simulink model "Grua_MC_R2_FFLimitado_06102026"  (R2025b)
settings: Solver=ode23t  StartTime=0.0  StopTime=628  MaxStep=T_s  RelTol=1e-4
InitFcn:
  | addpath(fileparts(get_param('Grua_MC_R2_FFLimitado_06102026','FileName')),'-begin');
  | run(fullfile(fileparts(get_param('Grua_MC_R2_FFLimitado_06102026','FileName')),'definir_buses_variadores.m'));
  | run(fullfile(fileparts(get_param('Grua_MC_R2_FFLimitado_06102026','FileName')),'parametros_ganancias_cascada_29072026.m'));
  | run(fullfile(fileparts(get_param('Grua_MC_R2_FFLimitado_06102026','FileName')),'configurar_modelo_final_hmi.m'));
  | run(fullfile(fileparts(get_param('Grua_MC_R2_FFLimitado_06102026','FileName')),'configurar_parametros_variadores.m'));
  | 
  | 
  | 
  | 
  | 
  | 
  | 
  | Pvis.Ts_viz=.04;Pvis.enable=true;Pvis.keepFigureOnTerminate=true;Pvis.hmi.captureFolder='D:\AyCD\Chat\Proyecto_grua\Prueba_Completa_MC_20261007\corrida_09';Pvis.hmi.fastDiagnostic=false;Pvis.hmi.testDriver=@operador_dos_traslados_v4;Pvis.hmi.renderPeriod=.20;
StopFcn:
  | guardar_prueba_completa;
undefined symbols (not defined in the file): b_cx, b_cy, b_hb, b_hEb, b_heq, b_t, b_tb, b_teq, b_tw, b_wu, g, H_c, HMI, i_h, i_t, J_heq, J_teq, K_cy, K_tw, k_wu, L_h0, l_hi, M_c_profile, M_s, M_t, MC_FF, nLevels0, omega_hmRATED, r_hd, r_td, slotBlock, T_hbMax, T_hEbMax, T_hmMax, T_s, T_s1, T_tbMax, T_tmMax, tau_hm, tau_tm, traj_duration, traj_x_start, traj_x_target, v_hmaxLoaded, v_hmaxUnloaded, x_tmax, x_tmin, Y_c0, Y_t0, Zbase
libraries: simulink x1, aerolibanimutils x1
(part 3 of 5)

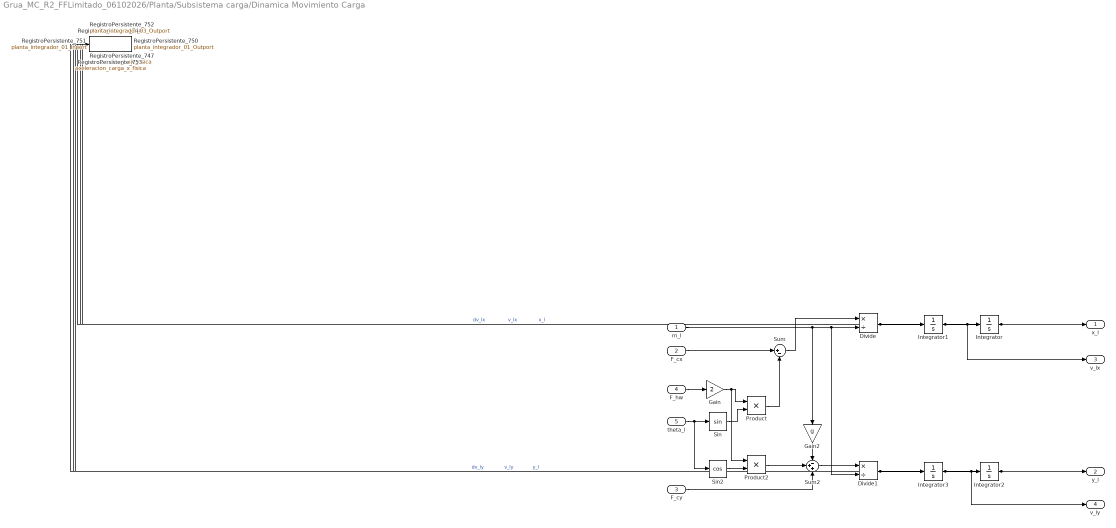
== system Grua_MC_R2_FFLimitado_06102026/Planta/Subsistema carga/Dinamica Movimiento Carga ==
  m_l : Inport
  F_cx : Inport  Port=2
  F_cy : Inport  Port=3
  F_hw : Inport  Port=4
  theta_l : Inport  Port=5
  Divide : Product  Inputs=*/
  Divide1 : Product  Inputs=*/
  Gain : Gain  Gain=2
  Gain2 : Gain  Gain=g
  Integrator : Integrator
  Integrator1 : Integrator
  Integrator2 : Integrator  InitialCondition=25
  Integrator3 : Integrator
  Product : Product
  Product2 : Product
  RegistroPersistente_746 : ToWorkspace  VariableName=diag_load_acc1  SaveFormat=Timeseries  SampleTime=-1
      settings: Decimation=10
  RegistroPersistente_747 : ToWorkspace  VariableName=aceleracion_izaje_fisica  SaveFormat=Timeseries  SampleTime=-1
      settings: Decimation=10
  RegistroPersistente_750 : ToWorkspace  VariableName=planta_integrador_01_Outport  SaveFormat=Timeseries  SampleTime=-1
      settings: Decimation=10
  RegistroPersistente_751 : ToWorkspace  VariableName=planta_integrador_01_Inport  SaveFormat=Timeseries  SampleTime=-1
      settings: Decimation=10
  RegistroPersistente_752 : ToWorkspace  VariableName=planta_integrador_03_Outport  SaveFormat=Timeseries  SampleTime=-1
      settings: Decimation=10
  RegistroPersistente_753 : ToWorkspace  VariableName=aceleracion_carga_x_fisica  SaveFormat=Timeseries  SampleTime=-1
      settings: Decimation=10
  Sin : Trigonometry
  Sin2 : Trigonometry  Operator=cos
  Sum : Sum  Inputs=|+-
  Sum2 : Sum  Inputs=-++
  x_l : Outport
  y_l : Outport  Port=2
  v_lx : Outport  Port=3
  v_ly : Outport  Port=4
  wires:
  Integrator/1 -> x_l/1, RegistroPersistente_750/1  "x_l"
  Integrator1/1 -> v_lx/1, Integrator/1, RegistroPersistente_751/1  "v_lx"
  Divide/1 -> Integrator1/1, RegistroPersistente_746/1  "dv_lx"
  Sum/1 -> Divide/1
  F_cx/1 -> Sum/1
  Gain/1 -> Product2/1, Product/1
  F_hw/1 -> Gain/1
  theta_l/1 -> Sin2/1, Sin/1
  Sin/1 -> Product/2
  Product/1 -> Sum/2
  Divide1/1 -> Integrator3/1, RegistroPersistente_747/1  "dv_ly"
  F_cy/1 -> Sum2/3
  m_l/1 -> Divide1/2, Divide/2, Gain2/1
  Integrator3/1 -> v_ly/1, Integrator2/1, RegistroPersistente_753/1  "v_ly"
  Integrator2/1 -> y_l/1, RegistroPersistente_752/1  "y_l"
  Sin2/1 -> Product2/2
  Product2/1 -> Sum2/2
  Gain2/1 -> Sum2/1
  Sum2/1 -> Divide1/1

== system Grua_MC_R2_FFLimitado_06102026/Planta/Subsistema carro/Dinamica Carro Traslacional ==
  F_tw : Inport
  F_hw : Inport  Port=2
  theta_l : Inport  Port=3
  Gain : Gain  Gain=1/M_t
  Gain1 : Gain  Gain=b_t
  Gain2 : Gain  Gain=2
  Integrator : Integrator
  Integrator1 : Integrator
  Product : Product
  RegistroPersistente_773 : ToWorkspace  VariableName=aceleracion_carro_fisica  SaveFormat=Timeseries  SampleTime=-1
      settings: Decimation=10
  RegistroPersistente_776 : ToWorkspace  VariableName=planta_integrador_05_Outport  SaveFormat=Timeseries  SampleTime=-1
      settings: Decimation=10
  RegistroPersistente_777 : ToWorkspace  VariableName=diag_xtrolley  SaveFormat=Timeseries  SampleTime=-1
      settings: Decimation=10
  Sin : Trigonometry
  Sum : Sum  Inputs=++-
  x_t : Outport
  v_t : Outport  Port=2
  wires:
  Sum/1 -> Gain/1
  Product/1 -> Gain2/1
  Gain/1 -> Integrator/1, RegistroPersistente_773/1  "ddx_t"
  Gain2/1 -> Sum/1  "ddx_t"
  Integrator1/1 -> x_t/1, RegistroPersistente_777/1  "x_t"
  F_tw/1 -> Sum/2
  Gain1/1 -> Sum/3
  Integrator/1 -> Gain1/1, v_t/1, Integrator1/1, RegistroPersistente_776/1  "v_t"
  Sin/1 -> Product/1
  F_hw/1 -> Product/2
  theta_l/1 -> Sin/1

== system Grua_MC_R2_FFLimitado_06102026/Planta/Subsistema carro/Dinamica Tambor Carro ==
  F_tw : Inport
  T_tm : Inport  Port=2
  T_tb : Inport  Port=3
  Gain3 : Gain  Gain=1/J_teq
  Gain4 : Gain  Gain=b_teq
  Gain5 : Gain  Gain=1/i_t
  Gain6 : Gain  Gain=r_td
  Gain7 : Gain  Gain=r_td
  Gain8 : Gain  Gain=r_td
  Integrator2 : Integrator
  Integrator3 : Integrator
  RegistroPersistente_788 : ToWorkspace  VariableName=planta_integrador_07_Inport  SaveFormat=Timeseries  SampleTime=-1
      settings: Decimation=10
  RegistroPersistente_792 : ToWorkspace  VariableName=diag_xdrum  SaveFormat=Timeseries  SampleTime=-1
      settings: Decimation=10
  RegistroPersistente_793 : ToWorkspace  VariableName=diag_vdrum  SaveFormat=Timeseries  SampleTime=-1
      settings: Decimation=10
  RegistroPersistente_794 : ToWorkspace  VariableName=planta_integrador_07_Outport  SaveFormat=Timeseries  SampleTime=-1
      settings: Decimation=10
  RegistroPersistente_795 : ToWorkspace  VariableName=planta_integrador_08_Outport  SaveFormat=Timeseries  SampleTime=-1
      settings: Decimation=10
  Sum1 : Sum  Inputs=++--
  x_td : Outport
  dx_td : Outport  Port=2
  theta_td : Outport  Port=3
  omega_td : Outport  Port=4
  wires:
  Gain3/1 -> Integrator2/1, RegistroPersistente_788/1  "ddtheta_td"
  Integrator2/1 -> omega_td/1, Gain4/1, Gain8/1, Integrator3/1, RegistroPersistente_794/1  "omega_td"
  Sum1/1 -> Gain3/1
  T_tb/1 -> Sum1/2
  Integrator3/1 -> Gain7/1, theta_td/1, RegistroPersistente_795/1  "theta_td"
  Gain6/1 -> Gain5/1  "T_tdl"
  Gain4/1 -> Sum1/4
  Gain5/1 -> Sum1/3  "ddtheta_td"
  T_tm/1 -> Sum1/1
  Gain7/1 -> x_td/1, RegistroPersistente_792/1  "x_td"
  Gain8/1 -> dx_td/1, RegistroPersistente_793/1  "dx_td"
  F_tw/1 -> Gain6/1

== system Grua_MC_R2_FFLimitado_06102026/Planta/Subsistema carro/Dinamica cable carro ==
  x_t : Inport
  dx_t : Inport  Port=2
  x_td : Inport  Port=3
  dx_td : Inport  Port=4
  Gain10 : Gain  Gain=b_tw
  Gain9 : Gain  Gain=K_tw
  Sum2 : Sum  Inputs=|+-
  Sum3 : Sum  Inputs=|+-
  Sum4 : Sum
  F_tw : Outport
  wires:
  x_t/1 -> Sum2/2
  Gain9/1 -> Sum4/1  "T_tdl"
  Sum4/1 -> F_tw/1  "F_tw"
  dx_t/1 -> Sum3/2
  dx_td/1 -> Sum3/1
  Sum2/1 -> Gain9/1
  Sum3/1 -> Gain10/1
  x_td/1 -> Sum2/1
  Gain10/1 -> Sum4/2  "T_tdl"

== system Grua_MC_R2_FFLimitado_06102026/Planta/Subsistema carro/Modelo Freno Operacion Carro ==
  BRK_t : Inport
  omega_tm : Inport  Port=2
  Constant : Constant  Value=0
  Gain : Gain  Gain=-b_tb
  RegistroPersistente_815 : ToWorkspace  VariableName=diag_brake_torque  SaveFormat=Timeseries  SampleTime=-1
      settings: Decimation=10
  Saturation : Saturate  UpperLimit=T_tbMax  LowerLimit=-T_tbMax
  Switch : Switch  Criteria=u2 > Threshold  SaturateOnIntegerOverflow=off  InputSameDT=off
  T_tb : Outport
  wires:
  Saturation/1 -> Switch/3
  omega_tm/1 -> Gain/1
  Switch/1 -> T_tb/1, RegistroPersistente_815/1
  Gain/1 -> Saturation/1
  Constant/1 -> Switch/1
  BRK_t/1 -> Switch/2

== system Grua_MC_R2_FFLimitado_06102026/Planta/Subsistema carro/Modulador de Torque Motor Drive Carro ==
  T_tm* : Inport
  Diferencia torque saturacion : Sum  Inputs=+-
  Gain : Gain  Gain=1/tau_tm
  Integrator : Integrator
  RegistroPersistente_819 : ToWorkspace  VariableName=aw_delta_torque_Nm  SaveFormat=Timeseries  SampleTime=-1
      settings: Decimation=10
  RegistroPersistente_820 : ToWorkspace  VariableName=planta_integrador_09_Inport  SaveFormat=Timeseries  SampleTime=-1
      settings: Decimation=10
  RegistroPersistente_821 : ToWorkspace  VariableName=planta_integrador_09_Outport  SaveFormat=Timeseries  SampleTime=-1
      settings: Decimation=10
  RegistroPersistente_822 : ToWorkspace  VariableName=torque_carro_limitado  SaveFormat=Timeseries  SampleTime=-1
      settings: Decimation=10
  Saturation : Saturate  UpperLimit=T_tmMax  LowerLimit=-T_tmMax
  Sum : Sum  Inputs=|+-
  T_tm : Outport
  Delta torque limite : Outport  Port=2
  wires:
  Integrator/1 -> Sum/2, T_tm/1, RegistroPersistente_821/1
  Gain/1 -> Integrator/1, RegistroPersistente_820/1
  Sum/1 -> Gain/1
  Saturation/1 -> Sum/1, Diferencia torque saturacion/1, RegistroPersistente_822/1  "T_tmlim*"
  T_tm*/1 -> Saturation/1, Diferencia torque saturacion/2
  Diferencia torque saturacion/1 -> Delta torque limite/1, RegistroPersistente_819/1

== system Grua_MC_R2_FFLimitado_06102026/Planta/Subsistema izaje/Calculo longitud l_h ==
  note: $\dot{l}_h(t)=-\frac{r_{hd}}{2}\omega_{hd}(t)$
  omega_hd : Inport
  Gain : Gain  Gain=-r_hd/2
  Integrator : Integrator  InitialCondition=l_hi
  RegistroPersistente_837 : ToWorkspace  VariableName=planta_integrador_10_Inport  SaveFormat=Timeseries  SampleTime=-1
      settings: Decimation=10
  RegistroPersistente_838 : ToWorkspace  VariableName=planta_integrador_10_Outport  SaveFormat=Timeseries  SampleTime=-1
      settings: Decimation=10
  l_h : Outport
  dl_h : Outport  Port=2
  wires:
  Integrator/1 -> l_h/1, RegistroPersistente_838/1  "l_h"
  omega_hd/1 -> Gain/1
  Gain/1 -> dl_h/1, Integrator/1, RegistroPersistente_837/1  "dl_h"

== system Grua_MC_R2_FFLimitado_06102026/Planta/Subsistema izaje/Dinamica Tambor Izaje ==
  T_hEb : Inport
  T_hm : Inport  Port=2
  F_hw : Inport  Port=3
  T_hb : Inport  Port=4
  Gain1 : Gain  Gain=r_hd
  Gain2 : Gain  Gain=1/i_h
  Gain3 : Gain  Gain=1/J_heq
  Gain4 : Gain  Gain=b_heq
  Gain5 : Gain  Gain=1/i_h
  Integrator2 : Integrator
  Integrator3 : Integrator
  RegistroPersistente_847 : ToWorkspace  VariableName=planta_integrador_11_Inport  SaveFormat=Timeseries  SampleTime=-1
      settings: Decimation=10
  RegistroPersistente_850 : ToWorkspace  VariableName=tambor_izaje_velocidad_angular  SaveFormat=Timeseries  SampleTime=-1
      settings: Decimation=10
  RegistroPersistente_851 : ToWorkspace  VariableName=planta_integrador_12_Outport  SaveFormat=Timeseries  SampleTime=-1
      settings: Decimation=10
  Sum1 : Sum  Inputs=+++--
  theta_hd : Outport
  omega_hd : Outport  Port=2
  wires:
  Gain3/1 -> Integrator2/1, RegistroPersistente_847/1  "ddtheta_hd"
  Integrator2/1 -> omega_hd/1, Gain4/1, Integrator3/1, RegistroPersistente_850/1  "omega_hd"
  Sum1/1 -> Gain3/1
  T_hb/1 -> Sum1/2
  T_hEb/1 -> Gain5/1  "T_hEb"
  Gain4/1 -> Sum1/5
  Gain5/1 -> Sum1/3
  T_hm/1 -> Sum1/1
  F_hw/1 -> Gain1/1
  Gain1/1 -> Gain2/1  "T_hdl"
  Gain2/1 -> Sum1/4
  Integrator3/1 -> theta_hd/1, RegistroPersistente_851/1  "theta_hd"

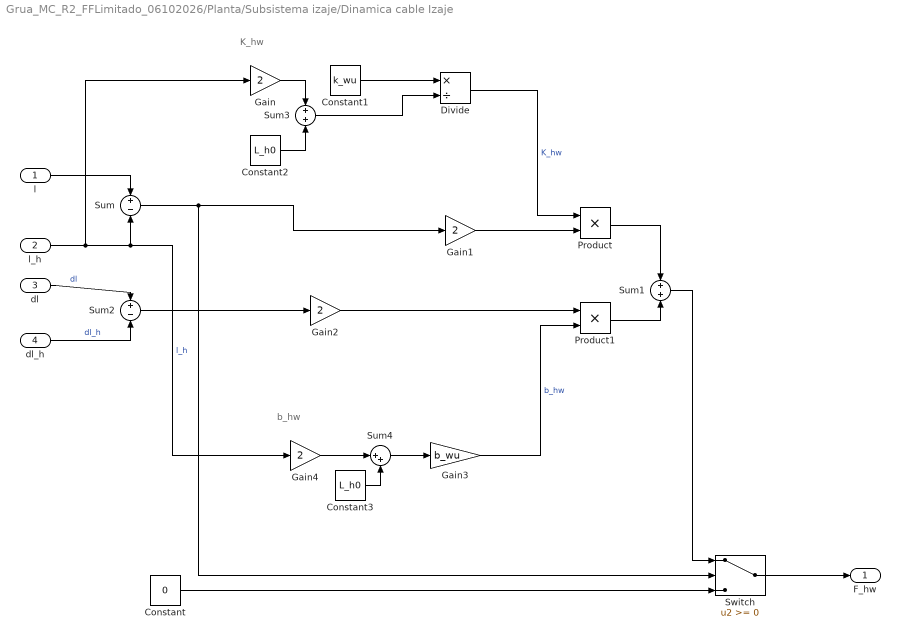
== system Grua_MC_R2_FFLimitado_06102026/Planta/Subsistema izaje/Dinamica cable Izaje ==
  note: b_hw
  note: K_hw
  l : Inport
  l_h : Inport  Port=2
  dl : Inport  Port=3
  dl_h : Inport  Port=4
  Constant : Constant  Value=0
  Constant1 : Constant  Value=k_wu
  Constant2 : Constant  Value=L_h0
  Constant3 : Constant  Value=L_h0
  Divide : Product  Inputs=*/
  Gain{,1..2,4} (4 alike) : Gain  Gain=2
  Gain3 : Gain  Gain=b_wu
  Product : Product
  Product1 : Product
  Sum : Sum  Inputs=+-
  Sum1 : Sum
  Sum2 : Sum  Inputs=+-
  Sum3 : Sum
  Sum4 : Sum  Inputs=|++
  Switch : Switch  SaturateOnIntegerOverflow=off  InputSameDT=off
  F_hw : Outport
  wires:
  Constant/1 -> Switch/3
  l/1 -> Sum/1
  l_h/1 -> Gain4/1, Sum/2, Gain/1  "l_h"
  Sum/1 -> Switch/2, Gain1/1
  Switch/1 -> F_hw/1
  Sum1/1 -> Switch/1
  Gain1/1 -> Product/2
  Product/1 -> Sum1/1
  Divide/1 -> Product/1  "K_hw"
  Gain3/1 -> Product1/2  "b_hw"
  dl/1 -> Sum2/1  "dl"
  dl_h/1 -> Sum2/2  "dl_h"
  Sum2/1 -> Gain2/1
  Gain2/1 -> Product1/1
  Product1/1 -> Sum1/2
  Sum3/1 -> Divide/2
  Constant1/1 -> Divide/1
  Constant2/1 -> Sum3/2
  Gain/1 -> Sum3/1
  Gain4/1 -> Sum4/1
  Sum4/1 -> Gain3/1
  Constant3/1 -> Sum4/2

== system Grua_MC_R2_FFLimitado_06102026/Planta/Subsistema izaje/Modelo Freno Emergencia de Izaje(Eje lento) ==
  omega_hd : Inport
  BRK_hE : Inport  Port=2
  Constant : Constant  Value=0
  Gain : Gain  Gain=-b_hEb
  Saturation : Saturate  UpperLimit=T_hEbMax  LowerLimit=-T_hEbMax
  Switch : Switch  Criteria=u2 > Threshold  SaturateOnIntegerOverflow=off  InputSameDT=off
  T_hEb : Outport
  wires:
  Saturation/1 -> Switch/3
  omega_hd/1 -> Gain/1
  Switch/1 -> T_hEb/1
  Gain/1 -> Saturation/1
  Constant/1 -> Switch/1
  BRK_hE/1 -> Switch/2

== system Grua_MC_R2_FFLimitado_06102026/Planta/Subsistema izaje/Modelo Freno Operacion de Izaje(Eje Rapido) ==
  BRK_h : Inport
  omega_hm : Inport  Port=2
  Constant : Constant  Value=0
  Gain : Gain  Gain=-b_hb
  RegistroPersistente_891 : ToWorkspace  VariableName=freno_operacion_izaje_torque  SaveFormat=Timeseries  SampleTime=-1
      settings: Decimation=10
  Saturation : Saturate  UpperLimit=T_hbMax  LowerLimit=-T_hbMax
  Switch : Switch  Criteria=u2 > Threshold  SaturateOnIntegerOverflow=off  InputSameDT=off
  T_hb : Outport
  wires:
  Saturation/1 -> Switch/3
  omega_hm/1 -> Gain/1
  Switch/1 -> T_hb/1, RegistroPersistente_891/1
  Gain/1 -> Saturation/1
  Constant/1 -> Switch/1
  BRK_h/1 -> Switch/2

== system Grua_MC_R2_FFLimitado_06102026/Planta/Subsistema izaje/Modulador de Torque Motor Drive Izaje ==
  T_hm* : Inport
  omega_hm : Inport  Port=2
  Calculo Torque Limite : Subsystem
  Gain : Gain  Gain=1/tau_hm
  Gain1 : Gain  Gain=-1
  Integrator : Integrator
  RegistroPersistente_905 : ToWorkspace  VariableName=planta_integrador_13_Inport  SaveFormat=Timeseries  SampleTime=-1
      settings: Decimation=10
  RegistroPersistente_907 : ToWorkspace  VariableName=planta_integrador_13_Outport  SaveFormat=Timeseries  SampleTime=-1
      settings: Decimation=10
  RegistroPersistente_908 : ToWorkspace  VariableName=Thm_sat  SaveFormat=Timeseries  SampleTime=-1
      settings: Decimation=10
  Saturation Dynamic : simulink/Discontinuities/Saturation Dynamic  OutMin=[]  OutMax=[]  OutDataTypeStr=Inherit: Same as second input  OutDataType=fixdt(1, 16)  OutScaling=2^-10  DoSatur=off
  Sum : Sum  Inputs=|+-
  T_hm : Outport
  wires:
  Gain/1 -> Integrator/1, RegistroPersistente_905/1
  Sum/1 -> Gain/1
  Integrator/1 -> T_hm/1, Sum/2, RegistroPersistente_907/1
  Saturation Dynamic/1 -> Sum/1, RegistroPersistente_908/1  "Thm_sat"
  T_hm*/1 -> Saturation Dynamic/2
  omega_hm/1 -> Calculo Torque Limite/1(omega_hm)
  Calculo Torque Limite/1(T_hmMax) -> Gain1/1, Saturation Dynamic/1
  Gain1/1 -> Saturation Dynamic/3

== system Grua_MC_R2_FFLimitado_06102026/Planta/Subsistema izaje/Modulador de Torque Motor Drive Izaje/Calculo Torque Limite ==
  omega_hm : Inport
  Abs omega : Abs  SaturateOnIntegerOverflow=off
  Constant2 : Constant
  Divide : Product  Inputs=*/
  Gain1 : Gain  Gain=T_hmMax
  Min : MinMax  Inputs=2
  Proteccion omega cero : Saturate  UpperLimit=inf  LowerLimit=1e-6
  RegistroPersistente_900 : ToWorkspace  VariableName=T_hmMax  SaveFormat=Timeseries  SampleTime=-1
      settings: Decimation=10
  Square : Math  Operator=square
  omega_hmRATED : Constant  Value=omega_hmRATED
  T_hmMax : Outport
  wires:
  omega_hmRATED/1 -> Divide/1
  Gain1/1 -> T_hmMax/1, RegistroPersistente_900/1  "T_hmMax"
  Min/1 -> Gain1/1
  Constant2/1 -> Min/2
  Square/1 -> Min/1
  Divide/1 -> Square/1
  omega_hm/1 -> Abs omega/1
  Abs omega/1 -> Proteccion omega cero/1
  Proteccion omega cero/1 -> Divide/2

== matlab function Grua_MC_R2_FFLimitado_06102026/Nivel 0 - Seguridad/Sensores de seguridad ==
  data: xT input; LST_MINU output; vT input; yH input; vH input; LST_MAXU output; LSH_MINU output; LSH_MAXU output; VH_MAX output
function [LST_MINU,LST_MAXU,LSH_MINU,LSH_MAXU,VH_MAX] = detectar(xT,vT,yH,vH)
%#codegen
LST_MINU = (xT <= -30.5) || (vT <= -4.6);
LST_MAXU = (xT >=  50.5) || (vT >=  4.6);
LSH_MINU = yH <= -20.5;
LSH_MAXU = yH >=  40.5;
VH_MAX = abs(vH) >= 3.45;
end

== stateflow chart Grua_MC_R2_FFLimitado_06102026/Nivel 0 - Seguridad/Automata de proteccion ==
  settings: updateMethod=DISCRETE  sampleTime=T_s0
  state SALTOS_EMERGENCIAS [parallel]
    settings: executionOrder=1
    state FUNCIONAMIENTO_NORMAL
      entry:
      EMERGENCIA=false;
      BRK_t=true;
      BRK_h=true;
      BRK_hE=true;
    state EMERGENCIA_IZAJE
      entry:
      EMERGENCIA=true;
      BRK_t=true;
      BRK_h=false;
      BRK_hE=false;
    state EMERGENCIA_CARRO
      entry:
      EMERGENCIA=true;
      BRK_t=false;
      BRK_h=true;
      BRK_hE=true;
    state EMERGENCIA_TOTAL
      entry:
      EMERGENCIA=true;
      BRK_t=false;
      BRK_h=false;
      BRK_hE=false;
    (default) -> SALTOS_EMERGENCIAS.FUNCIONAMIENTO_NORMAL
    SALTOS_EMERGENCIAS.FUNCIONAMIENTO_NORMAL -> EMERGENCIA_CARRO [order 3] : [hasChangedTo(LST_MAXU,1) || hasChangedTo(LST_MINU,1)]
    SALTOS_EMERGENCIAS.FUNCIONAMIENTO_NORMAL -> EMERGENCIA_IZAJE [order 2] : [hasChangedTo(LSH_MAXU,1) || hasChangedTo(LSH_MINU,1) || hasChangedTo(VH_MAX,1)]
    EMERGENCIA_CARRO -> SALTOS_EMERGENCIAS.FUNCIONAMIENTO_NORMAL [order 2] : [~BOTON_EMERGENCIA && ~LST_MAXU && ~LST_MINU && hasChangedTo(REINICIO,1)]
    EMERGENCIA_IZAJE -> SALTOS_EMERGENCIAS.FUNCIONAMIENTO_NORMAL [order 2] : [~BOTON_EMERGENCIA && ~LSH_MAXU && ~LSH_MINU && ~VH_MAX && hasChangedTo(REINICIO,1)]
    SALTOS_EMERGENCIAS.FUNCIONAMIENTO_NORMAL -> EMERGENCIA_TOTAL [order 1] : [BOTON_EMERGENCIA || PARADA_EMERGENCIA_WD]
    EMERGENCIA_TOTAL -> SALTOS_EMERGENCIAS.FUNCIONAMIENTO_NORMAL : [~BOTON_EMERGENCIA && ~PARADA_EMERGENCIA_WD && ~LST_MAXU && ~LST_MINU && ~LSH_MAXU && ~LSH_MINU && ~VH_MAX && hasChangedTo(REINICIO,1)]
    EMERGENCIA_CARRO -> EMERGENCIA_TOTAL [order 1] : [hasChangedTo(LSH_MAXU,1) || hasChangedTo(LSH_MINU,1) || hasChangedTo(VH_MAX,1) || BOTON_EMERGENCIA || PARADA_EMERGENCIA_WD]
    EMERGENCIA_IZAJE -> EMERGENCIA_TOTAL [order 1] : [hasChangedTo(LST_MAXU,1) || hasChangedTo(LST_MINU,1) || BOTON_EMERGENCIA || PARADA_EMERGENCIA_WD]
  state WATCHDOG [parallel]
    settings: executionOrder=2
    state FUNCIONAMIENTO_NORMAL
      entry:
      PARADA_EMERGENCIA_WD=false;
    state FALLO_WD
      entry:
      PARADA_EMERGENCIA_WD=true;
    (default) -> WATCHDOG.FUNCIONAMIENTO_NORMAL
    FALLO_WD -> WATCHDOG.FUNCIONAMIENTO_NORMAL : [hasChangedTo(REINICIO,1)]
    WATCHDOG.FUNCIONAMIENTO_NORMAL -> WATCHDOG.FUNCIONAMIENTO_NORMAL [order 2] : [hasChanged(pulso_WD)]
    WATCHDOG.FUNCIONAMIENTO_NORMAL -> FALLO_WD [order 1] : [after(TiempoMaxWD, sec)]
  data: pulso_WD input boolean; REINICIO input boolean; BRK_h output boolean; BRK_hE output boolean; BRK_t output boolean; EMERGENCIA output boolean; LST_MINU input boolean; LST_MAXU input boolean; LSH_MINU input boolean; LSH_MAXU input boolean; TiempoMaxWD input double =10; BOTON_EMERGENCIA input boolean; VH_MAX input boolean; PARADA_EMERGENCIA_WD output boolean

== matlab function Grua_MC_R2_FFLimitado_06102026/MASS_latch_pick ==
  settings: updateMethod=DISCRETE  sampleTime=0.001
  data: profileMass input; mass output; loaded input
function mass = latchPickedMass(profileMass,loaded)
%#codegen
persistent heldMass previousLoaded
if isempty(heldMass)
    heldMass=0.0; previousLoaded=false;
end
isLoaded=loaded>=0.5;
if isLoaded && ~previousLoaded
    heldMass=max(0.0,profileMass);
elseif ~isLoaded
    heldMass=0.0;
end
mass=heldMass; previousLoaded=isLoaded;
end

== matlab function Grua_MC_R2_FFLimitado_06102026/Motion Controller/MC Izaje ==
  settings: updateMethod=DISCRETE  sampleTime=T_s
  data: s input Bus: MCFF_Sensors; torque output; r input Bus: MCFF_References; est input Bus: MCFF_HoistState; p input Bus: MCFF_Parameters; d output Bus: MCFF_HoistDiagnostics
function [torque,d]=fcn(s,r,est,p)
%#codegen
% Variador de izaje. No implementa ninguna funcion del automata.
[torque,ev,z1,z2,P,D,I,ff]=controlador_izaje_mc_r2( ...
 s.force,-r.hoistVelocityRef,est.lengthRate,-r.hoistAccelerationRef,p);
d=struct('torque_izaje_consigna_controlador',torque,'mc_hoist_velocity_error',ev, ...
 'mc_hoist_integral1',z1,'mc_hoist_integral2',z2,'mc_hoist_P',P, ...
 'mc_hoist_D',D,'mc_hoist_I',I,'mc_hoist_FF',ff);
end
function [torque,errorVelocity,z1,z2,pTerm,dTerm,iTerm,ff]= ...
 controlador_izaje_mc_r2(force,vRef,vMeasured,aRef,p)
%#codegen
% Doble integracion Tustin de R2, sin seleccion por modo ni AW adicional.
persistent firstIntegral secondIntegral previousError previousFirst
if isempty(firstIntegral)
 firstIntegral=0.0;secondIntegral=0.0;previousError=0.0;previousFirst=0.0;
end
errorVelocity=vRef-vMeasured;
firstIntegral=(p.Ts/2)*(previousError+errorVelocity)+firstIntegral;
secondIntegral=(p.Ts/2)*(previousFirst+firstIntegral)+secondIntegral;
z1=firstIntegral;z2=secondIntegral;
pTerm=p.Khp*z1;dTerm=p.Khd*errorVelocity;iTerm=p.Khi*z2;
feedback=(iTerm+pTerm)+dTerm;
forceTerm=(-p.r_hd/p.i_h)*force;
ff=(-p.r_hd/p.i_h)*(p.M_EQh*aRef+p.b_EQh*vRef);
torque=ff+(feedback-forceTerm);
previousError=errorVelocity;previousFirst=firstIntegral;
end

== matlab function Grua_MC_R2_FFLimitado_06102026/Motion Controller/MC Carro ==
  settings: updateMethod=DISCRETE  sampleTime=T_s
  data: s input Bus: MCFF_Sensors; torque output; r input Bus: MCFF_References; c input Bus: MCFF_Commands; drive input Bus: MCFF_DriveFeedback; est input Bus: MCFF_TrolleyState; hoist input Bus: MCFF_HoistState; p input Bus: MCFF_Parameters; sw output; d output Bus: MCFF_TrolleyDiagnostics
function [torque,sw,d]=fcn(s,r,c,drive,est,hoist,p)
%#codegen
% Variador de carro. Estimaciones recibidas del estimador interno del MC.
persistent ff gain
if isempty(gain),ff=0.0;gain=0.0;end
omega=est.omegaDrum;
k=2.0*sqrt(p.gravity*hoist.length); anticipationGain=2.0*sqrt(9.80665*max(1.0,hoist.length));
thetaEff=double(c.E)*s.theta;
feedback=k*(thetaEff-0.0);
thetaRef=atan2(-r.aRef,p.gravity);
if ~c.E || ~c.brakeOpen
 ff=0.0;gain=0.0;sw=0.0;feedbackUsed=0.0;anticipationUsed=0.0;
else
 gain=min(1.0,gain+max(1e-6,p.Ts)/p.swayOnTime);
 target=-anticipationGain*thetaRef;
 h=max(1e-6,p.Ts);
 ff=ff+min(p.swayFFRate*h,max(-p.swayFFRate*h,target-ff));
 anticipation=ff;
 feedbackUsed=gain*feedback;anticipationUsed=gain*anticipation;
 sw=min(3.2,max(-3.2,feedbackUsed+anticipationUsed));
end
vBase=(r.vRef+sw)+r.swTransfer;
[torque,vRaw,vCmd,vObs,I,pTerm,iTerm,aRaw,aCmd,ev,deltaA,deltaAPrevious, ...
 deltaATorque,deltaATotal,awCorrection,uI]=controlador_carro_mc_r2( ...
 s.force,omega,vBase,r.xRef,r.aRef,est.x,s.theta,drive.deltaTorqueDelayed,p);
d=struct('diag_torque_unsat',torque,'diag_vcmd',vRaw,'diag_vcmd_applied',vCmd, ...
 'diag_vobs',vObs,'diag_integral',I,'diag_p',pTerm,'diag_i',iTerm,'diag_acmd',aRaw, ...
 'diag_acmd_applied',aCmd,'diag_ev',ev,'aw_delta_a_limite',deltaA, ...
 'aw_delta_a_limite_memoria',deltaAPrevious,'aw_delta_a_torque',deltaATorque, ...
 'aw_delta_a_total',deltaATotal,'aw_correccion_integrador',awCorrection, ...
 'mc_integrator_input',uI,'antisway_correccion_aplicada',sw, ...
 'sw_feedback_comun',feedbackUsed,'sw_anticipacion_comun',anticipationUsed, ...
 'sw_habilitacion_comun',gain,'diag_sw_unsat',feedback,'diag_sw_gain',k, ...
 'angulo_referencia',thetaRef,'diag_aff',r.aRef,'diag_xref_input',r.xRef, ...
 'diag_vref_input',r.vRef,'diag_aref_input',r.aRef,'diag_xencoder',est.x, ...
 'diag_omega_observer',omega,'diag_theta_medida',s.theta,'diag_theta_eff',thetaEff, ...
 'diag_brake_supervisor',double(c.brakeOpen));
end
function [torque,vRaw,vCmd,vObs,I,pTerm,iTerm,aRaw,aCmd,ev, ...
 deltaA,deltaAPrevious,deltaATorque,deltaATotal,awCorrection,uI]= ...
 controlador_carro_mc_r2(force,omega,vBase,xRef,aRef,x,theta,deltaTorque,p)
%#codegen
% N2 de R2: PI Tustin limitado, AW de aceleracion y torque con demora 1 ms.
% El regulador no recibe modo, enable de eje ni reset; N0 autoriza el par.
persistent integralState previousDeltaA
if isempty(integralState)
 integralState=0.0;previousDeltaA=0.0;
end
vObs=p.r_td*omega;
vRaw=vBase+p.Kx*(xRef-x);
vCmd=min(p.vmax,max(-p.vmax,vRaw));
ev=vCmd-vObs;
deltaAPrevious=previousDeltaA;
deltaATorque=(p.i_t/(p.r_td*p.M_EQt))*deltaTorque;
deltaATotal=deltaAPrevious+deltaATorque;
awCorrection=(1/p.Ki)*deltaATotal;
uI=ev+awCorrection;
% IC=0 es el estado X; la salida incluye el medio paso de entrada actual.
I=min(p.Imax,max(-p.Imax,integralState+p.Ts/2*uI));
% El bloque original limita salida Y y estado X por separado en Tustin.
% Esto permite salir del limite en el primer medio paso de signo contrario.
integralState=min(p.Imax,max(-p.Imax,I+p.Ts/2*uI));
pTerm=p.Kp*ev;iTerm=p.Ki*I;
aRaw=aRef+(pTerm+iTerm);
aCmd=min(p.amax,max(-p.amax,aRaw));
deltaA=aCmd-aRaw;
% Conservar la estructura de operaciones del Computed Torque de R2.
friction=(p.b_EQt/p.M_EQt)*vObs;
horizontal=(2/p.M_EQt)*(force*sin(theta));
torque=((p.r_td*p.M_EQt)/p.i_t)*((friction+aCmd)-horizontal);
previousDeltaA=deltaA;
end

== matlab function Grua_MC_R2_FFLimitado_06102026/Motion Controller/Estimadores ==
  settings: updateMethod=DISCRETE  sampleTime=T_s
  data: s input Bus: MCFF_Sensors; cart output Bus: MCFF_TrolleyState; p input Bus: MCFF_Parameters; hoist output Bus: MCFF_HoistState
function [cart,hoist]=fcn(s,p)
%#codegen
% Dos observadores Tustin de encoders, independientes de referencias y modos.
persistent qt wt qh wh previousT previousH started
if isempty(qt)
 qt=0.0;wt=0.0;qh=0.0;wh=0.0;previousT=0.0;previousH=0.0;started=false;
end
ut=s.motorAngleT/p.i_t;uh=s.motorAngleH/p.i_h;
if started
 [qt,wt]=actualizar_observador_encoder(qt,wt,previousT,ut,p);
 [qh,wh]=actualizar_observador_encoder(qh,wh,previousH,uh,p);
else
 started=true;
end
previousT=ut;previousH=uh;
cart=struct('x',p.r_td*ut,'omegaDrum',wt,'velocity',p.r_td*wt,'observerAngle',qt);
hoist=struct('length',p.length0-(p.r_hd/2)*uh,'lengthRate',(p.r_hd/(-2))*wh, ...
 'omegaDrum',wh,'observerAngle',qh);
end
function [qNext,wNext]=actualizar_observador_encoder(q,w,uPrevious,u,p)
%#codegen
% Trapezoidal: x[n]=Ad*x[n-1]+Bd*(u[n-1]+u[n]).
% La primera muestra y la IC=0 se manejan en el propietario del estado.
qNext=(p.obsA11*q+p.obsA12*w)+p.obsB1*(uPrevious+u);
wNext=(p.obsA21*q+p.obsA22*w)+p.obsB2*(uPrevious+u);
end

== matlab function Grua_MC_R2_FFLimitado_06102026/Consigna Izaje ==
  data: lh_ref output; dlh_ref output; t input; ddlh_ref output; done output
function [lh_ref, dlh_ref, ddlh_ref, done] = trayectoria_lh_quintica(t)
%#codegen
% Trayectoria suave para longitud de cable l_h.
%
% Tramo 1:
%   l_h: 20 m -> 34 m
%   inicia en t = 15 s
%
% Tramo 2:
%   l_h: 34 m -> 29 m
%   inicia en t = 45 s
%
% Salidas:
%   lh_ref   : referencia de longitud [m]
%   dlh_ref  : velocidad de longitud [m/s]
%   ddlh_ref : aceleración de longitud [m/s^2]
%   done     : true cuando terminó toda la secuencia

% Parámetros tramo 1: bajar / desenrollar
lh0_1   = 20.0;     % [m]
lhf_1   = 26.5;     % [m]
t_ini_1 = 15.0;     % [s]
Tmov_1  = 12.0;     % [s]

% Parámetros tramo 2: subir / enrollar 5 m
lh0_2   = lhf_1;    % [m]
lhf_2   = lhf_1 - 5.0;  % [m]
t_ini_2 = 28.0;     % [s]
Tmov_2  = 8.0;      % [s]

% Antes del primer movimiento
if t < t_ini_1
    lh_ref   = lh0_1;
    dlh_ref  = 0.0;
    ddlh_ref = 0.0;
    done     = false;
    return;
end

% Tramo 1
if t < t_ini_1 + Tmov_1
    [lh_ref, dlh_ref, ddlh_ref] = tramo_quintico(t, t_ini_1, Tmov_1, lh0_1, lhf_1);
    done = false;
    return;
end

% Espera entre tramo 1 y tramo 2
if t < t_ini_2
    lh_ref   = lhf_1;
    dlh_ref  = 0.0;
    ddlh_ref = 0.0;
    done     = false;
    return;
end

% Tramo 2
if t < t_ini_2 + Tmov_2
    [lh_ref, dlh_ref, ddlh_ref] = tramo_quintico(t, t_ini_2, Tmov_2, lh0_2, lhf_2);
    done = false;
    return;
end

% Después de terminar todo
lh_ref   = lhf_2;
dlh_ref  = 0.0;
ddlh_ref = 0.0;
done     = true;

end

function [lh, dlh, ddlh] = tramo_quintico(t, t_ini, Tmov, lh0, lhf)
% Trayectoria quintica normalizada entre lh0 y lhf.

tau = (t - t_ini) / Tmov;

s   = 10*tau^3 - 15*tau^4 + 6*tau^5;
ds  = 30*tau^2 - 60*tau^3 + 30*tau^4;
dds = 60*tau - 180*tau^2 + 120*tau^3;

Dlh = lhf - lh0;

lh   = lh0 + Dlh * s;
dlh  = Dlh * ds / Tmov;
ddlh = Dlh * dds / (Tmov^2);

end
